simulink library "HEV_Battery_Det_Lib"  (R2017a)
settings: Solver=ode45  StartTime=0.0  StopTime=0.1  RelTol=1e-3  EnableMultiTasking=on
undefined symbols (not defined in the file): BCell_R, HEV_Param, Hydride, Metal, Nickel
libraries: fl_lib x48, nesl_utility x32, Battery_Cell_Det x10, powerlib x8, elec_lib x3, HEV_Battery_Det_Lib x1, Capacitors_lib x1, electricdrivelib x1
Description:
  | Copyright 2014-2017 The MathWorks, Inc.
settings Model: Creator=smiller  LastModifiedBy=smiller
settings DataIOCC: LimitDataPoints=on  SaveFormat=Array  SignalLoggingSaveFormat=ModelDataLogs
settings OptimizationCC: ExpressionDepthLimit=2147483647  LifeSpan=inf
settings DebuggingCC: UnderspecifiedInitializationDetection=Classic  MergeDetectMultiDrivingBlocksExec=none  SolverPrmCheckMsg=warning  FcnCallInpInsideContextMsg=warning  AllowSymbolicDim=off  StateNameClashWarn=warning  SFUnexpectedBacktrackingDiag=warning  SFNoUnconditionalDefaultTransitionDiag=warning  SFExecutionAtInitializationDiag=none
settings HardwareCC: ProdBitPerPointer=32  ProdBitPerSizeT=32  ProdBitPerPtrDiffT=32  ProdLargestAtomicFloat=None  ProdIntDivRoundTo=Undefined  ProdEndianess=Unspecified  ProdWordSize=32  ProdHWDeviceType=32-bit Generic
settings ModelReferenceCC: PropagateSignalLabelsOutOfModel=off
settings GRTTargetCC: TargetLangStandard=C89/C90 (ANSI)  GeneratePreprocessorConditionals=Disable all  CombineOutputUpdateFcns=off  GRTInterface=on
settings ConfigComp: CovMetricSettings=dw  CovHtmlReporting=on  CovSaveCumulativeToWorkspaceVar=on  CovSaveSingleToWorkspaceVar=on  CovExternalEMLEnable=off  CovSFcnEnable=off

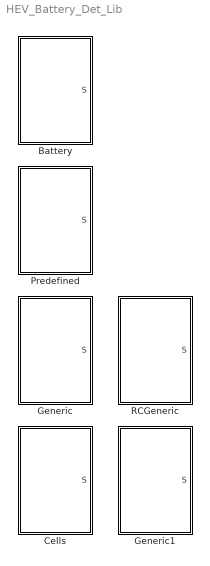
== system HEV_Battery_Det_Lib ==
  Battery : Subsystem  BlockChoice=Generic
      mask init:
      | %disp('Battery Mask Init');
      | %Configure_HEV_Simulation;
      settings: TemplateBlock=self  MemberBlocks=Generic,Predefined
  Cells : Subsystem
      mask Display:
      | image(imread('HEV_Battery_Cells_IMAGE.jpg'));
      | port_label('LConn',1,'+');
      | port_label('LConn',2,'-');
      | port_label('output',1,'S');
  Generic : Subsystem
      mask Display:
      | image(imread('HEV_Battery_Custom_IMAGE.jpg'));
      | port_label('LConn',1,'+');
      | port_label('LConn',2,'-');
      | port_label('output',1,'S');
  Generic1 : Subsystem
      mask Display:
      | image(imread('HEV_Battery_Generic_IMAGE.jpg'));
      | port_label('LConn',1,'+');
      | port_label('LConn',2,'-');
      | port_label('output',1,'S');
  Predefined : Subsystem
      mask Display:
      | image(imread('HEV_Battery_Detailed_IMAGE.jpg'));
      | port_label('LConn',1,'+');
      | port_label('LConn',2,'-');
      | port_label('output',1,'S');
  RCGeneric : Subsystem
      mask Display:
      | image(imread('HEV_Battery_GenericRC_IMAGE.jpg'));
      | port_label('LConn',1,'+');
      | port_label('LConn',2,'-');
      | port_label('output',1,'S');

== system HEV_Battery_Det_Lib/Battery ==
  Generic : HEV_Battery_Det_Lib/Generic  SystemSampleTime=-1
  + : PMIOPort  Port=1  Side=Left
  - : PMIOPort  Port=2  Side=Left
  S : Outport
  wires:
  Generic/1 -> S/1
  connections:
  Generic/LConn1 -- +/RConn1
  Generic/LConn2 -- -/RConn1

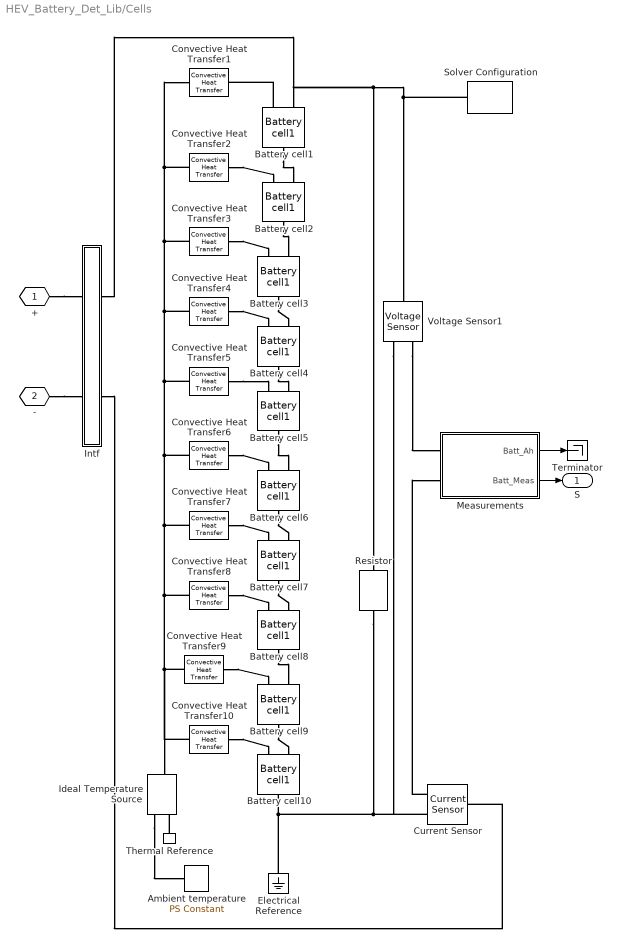
== system HEV_Battery_Det_Lib/Cells ==
  Ambient temperature : fl_lib/Physical Signals/Sources/PS Constant  constant=273+25
  Battery cell{1..10} (10 alike) : Battery_Cell_Det/Battery cell1  SystemSampleTime=-1
  Convective Heat Transfer{1..10} (10 alike) : fl_lib/Thermal/Thermal Elements/Convective Heat Transfer  area=HEV_Param.Battery_Cell.Area m^2  heat_tr_coeff=HEV_Param.Battery_Cell.Rtheta W/(m^2 *K)  Q_specify=off  Q_priority=High  Q=0 J/s  Q_nominal_specify=off  Q_nominal_unit=J/s  Q_nominal_value=1  T_specify=off  T_priority=High  T=0 K  T_nominal_specify=off  T_nominal_unit=K  T_nominal_value=1
  Current Sensor : fl_lib/Electrical/Electrical Sensors/Current Sensor
  Electrical Reference : fl_lib/Electrical/Electrical Elements/Electrical Reference
  Ideal Temperature Source : fl_lib/Thermal/Thermal Sources/Ideal Temperature Source
      settings: SourceProductName=Simscape  SourceProductBaseCode=SS
  Intf : Subsystem  mask(Power Systems ST - Simscape Interface Element){T=100000}
      mask prompts: T "Pole in Transfer Function"
      mask help:
      | Ideal transformer between a Simscape Power Systems ST circuit and a Simscape circuit.
      |
      | The Voltage across the two terminal pairs are equal and the current flowing through the two branches are equal.
      |
      | The coupling has a transfer function and you need to set the pole in the transfer function.
      mask Display:
      | %color('red');
      | %plot([0.3 0.7],[0.775 0.775]);
      | port_label('LConn', 1,'SPS1')
      | port_label('RConn', 1,'SS1')
      | color('black');
      | %plot([0.3 0.7],[0.225 0.225]);
      | port_label('LConn', 2,'SPS2')
      | port_label('RConn', 2,'SS2')
      | %color('green')
      | %text(0.05,0.5,'I Src');
      | %color('blue')
      | %text(0.75,0.5,'V Src');
  Measurements : Subsystem
  Resistor : fl_lib/Electrical/Electrical Elements/Resistor  R=BCell_R Ohm  i_specify=off  i_priority=High  i=0 A  i_nominal_specify=off  i_nominal_unit=A  i_nominal_value=1  v_specify=off  v_priority=High  v=0 V  v_nominal_specify=off  v_nominal_unit=V  v_nominal_value=1
  Solver Configuration : nesl_utility/Solver Configuration  PhysicalDomain=network_engine_domain  SubClassName=solver  LeftPortType=input  RightPortType=generic  Accelerate=off  Tones=[]  Harmonics=[]  SimulateNoise=off  Profile=off  UseLocalSampling=off  EnableSwitchedLinearOptims=on  FrequencyDomain=off  UseCCode=off  RelTol=0.001  AbsTol=1e-06  MinStep=1e-09  ToWorkspace=off  RevertToSquareIcSolve=off  NumHomotopyIterations=100  PhasorMode=off  PhasorModeNumHarmonics=1  OverrideAbsTol=off  DoDC=off  ResidualTolerance=1e-9  UseLocalSolver=off  LocalSolverChoice=NE_BACKWARD_EULER_ADVANCER  LocalSolverSampleTime=.001  DoFixedCost=off  MaxNonlinIter=3  MaxModeIter=2  LinearAlgebra=Sparse  DelaysMemoryBudget=1024  AutomaticFiltering=on  FilteringTimeConstant=0.001
  Terminator : Terminator
  Thermal Reference : fl_lib/Thermal/Thermal Elements/Thermal Reference
  Voltage Sensor1 : fl_lib/Electrical/Electrical Sensors/Voltage Sensor
  + : PMIOPort  Tag=PMCPort  Port=1  Side=Left
  - : PMIOPort  Tag=PMCPort  Port=2  Side=Left
  S : Outport
  wires:
  Measurements/2(Batt_Meas) -> S/1
  Measurements/1(Batt_Ah) -> Terminator/1
  connections:
  Voltage Sensor1/RConn1 -- Measurements/LConn1
  Current Sensor/RConn1 -- Measurements/LConn2
  Intf/RConn2 -- Current Sensor/LConn1
  Voltage Sensor1/RConn2 -- Current Sensor/RConn2 -- Battery cell10/RConn1 -- Electrical Reference/LConn1 -- Resistor/RConn1
  Convective Heat Transfer9/LConn1 -- Convective Heat Transfer10/LConn1 -- Ideal Temperature Source/LConn1 -- Convective Heat Transfer8/LConn1 -- Convective Heat Transfer7/LConn1 -- Convective Heat Transfer6/LConn1 -- Convective Heat Transfer5/LConn1 -- Convective Heat Transfer4/LConn1 -- Convective Heat Transfer3/LConn1 -- Convective Heat Transfer2/LConn1 -- Convective Heat Transfer1/LConn1
  Battery cell1/LConn2 -- Intf/RConn1 -- Voltage Sensor1/LConn1 -- Solver Configuration/RConn1 -- Resistor/LConn1
  Convective Heat Transfer9/RConn1 -- Battery cell9/LConn1
  Battery cell8/RConn1 -- Battery cell9/LConn2
  Convective Heat Transfer8/RConn1 -- Battery cell8/LConn1
  Convective Heat Transfer7/RConn1 -- Battery cell7/LConn1
  Battery cell7/RConn1 -- Battery cell8/LConn2
  Convective Heat Transfer6/RConn1 -- Battery cell6/LConn1
  Battery cell6/RConn1 -- Battery cell7/LConn2
  Battery cell5/RConn1 -- Battery cell6/LConn2
  Convective Heat Transfer5/RConn1 -- Battery cell5/LConn1
  Battery cell4/RConn1 -- Battery cell5/LConn2
  Convective Heat Transfer4/RConn1 -- Battery cell4/LConn1
  Battery cell3/RConn1 -- Battery cell4/LConn2
  Convective Heat Transfer3/RConn1 -- Battery cell3/LConn1
  Battery cell2/RConn1 -- Battery cell3/LConn2
  Battery cell9/RConn1 -- Battery cell10/LConn2
  Convective Heat Transfer2/RConn1 -- Battery cell2/LConn1
  Convective Heat Transfer10/RConn1 -- Battery cell10/LConn1
  Battery cell1/RConn1 -- Battery cell2/LConn2
  Battery cell1/LConn1 -- Convective Heat Transfer1/RConn1
  Ideal Temperature Source/RConn1 -- Ambient temperature/RConn1
  Thermal Reference/LConn1 -- Ideal Temperature Source/RConn2
  +/RConn1 -- Intf/LConn1
  -/RConn1 -- Intf/LConn2

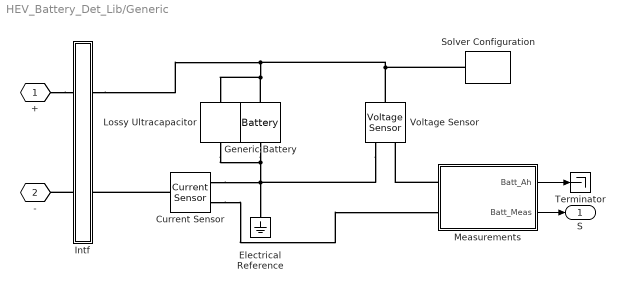
== system HEV_Battery_Det_Lib/Generic ==
  Current Sensor : fl_lib/Electrical/Electrical Sensors/Current Sensor
  Electrical Reference : fl_lib/Electrical/Electrical Elements/Electrical Reference
  Generic Battery : elec_lib/Sources/Battery  Vnom=HEV_Param.Battery_Sys.Nominal_Voltage V  R1=HEV_Param.Battery_Sys.Internal_Resistance Ohm  prm_AH=2  AH=HEV_Param.Battery_Sys.Rated_Capacity hr*A  V1=HEV_Param.Battery_Sys.Expn_Voltage V  AH1=HEV_Param.Battery_Sys.Expn_Charge hr*A  prm_R2=1  R2=2e+3 Ohm  prm_fade=1  N_fade=100  AH_fade=45 hr*A  R1_fade=2.02 Ohm  V1_fade=10.35 V  i_specify=off  i_priority=None  i=0 A  i_nominal_specify=off  i_nominal_unit=A  i_nominal_value=1  v_specify=off  v_priority=None  v=0 V  v_nominal_specify=off  v_nominal_unit=V  v_nominal_value=1  charge_specify=on  charge_priority=High  charge=HEV_Param.Battery_Sys.Initial_Charge hr*A  charge_nominal_specify=off  charge_nominal_unit=hr*A  charge_nominal_value=1  num_cycles_specify=off  num_cycles_priority=High  num_cycles=0  num_cycles_nominal_specify=off  num_cycles_nominal_unit=1  num_cycles_nominal_value=1  thermal_mass=30000 J/K  Tmeas=298.15 K  Vnom_T2=12 V  R1_T2=2.2 Ohm  V1_T2=11.4 V  R2_T2=2200 Ohm  Tmeas2=273.15 K  temperature_specify=off  temperature_priority=High  temperature=298.15 K  temperature_nominal_specify=off  temperature_nominal_unit=K  temperature_nominal_value=1
      settings: SourceProductName=Simscape Electronics  SourceProductBaseCode=SN
  Intf : Subsystem  mask(Power Systems ST - Simscape Interface Element){T=100000}
      mask prompts: T "Pole in Transfer Function"
      mask help:
      | Ideal transformer between a Simscape Power Systems ST circuit and a Simscape circuit.
      |
      | The Voltage across the two terminal pairs are equal and the current flowing through the two branches are equal.
      |
      | The coupling has a transfer function and you need to set the pole in the transfer function.
      mask Display:
      | %color('red');
      | %plot([0.3 0.7],[0.775 0.775]);
      | port_label('LConn', 1,'SPS1')
      | port_label('RConn', 1,'SS1')
      | color('black');
      | %plot([0.3 0.7],[0.225 0.225]);
      | port_label('LConn', 2,'SPS2')
      | port_label('RConn', 2,'SS2')
      | %color('green')
      | %text(0.05,0.5,'I Src');
      | %color('blue')
      | %text(0.75,0.5,'V Src');
  Lossy Ultracapacitor : Capacitors_lib/Lossy Ultracapacitor  C0=HEV_Param.UltraCapacitor.Nominal_Capacitance F  Cv=HEV_Param.UltraCapacitor.Rate_C_V F/V  R=HEV_Param.UltraCapacitor.Series_R Ohm  Rd=HEV_Param.UltraCapacitor.Self_Discharge_R Ohm  i_specify=off  i_priority=High  i=0 A  i_nominal_specify=off  i_nominal_unit=A  i_nominal_value=1  vc_specify=off  vc_priority=High  vc=0 V  vc_nominal_specify=off  vc_nominal_unit=V  vc_nominal_value=1
  Measurements : Subsystem
  Solver Configuration : nesl_utility/Solver Configuration  PhysicalDomain=network_engine_domain  SubClassName=solver  LeftPortType=input  RightPortType=generic  Accelerate=off  Tones=[]  Harmonics=[]  SimulateNoise=off  Profile=off  UseLocalSampling=off  EnableSwitchedLinearOptims=on  FrequencyDomain=off  UseCCode=off  RelTol=0.001  AbsTol=1e-06  MinStep=1e-09  ToWorkspace=off  RevertToSquareIcSolve=off  NumHomotopyIterations=100  PhasorMode=off  PhasorModeNumHarmonics=1  OverrideAbsTol=off  DoDC=off  ResidualTolerance=1e-9  UseLocalSolver=off  LocalSolverChoice=NE_BACKWARD_EULER_ADVANCER  LocalSolverSampleTime=.001  DoFixedCost=off  MaxNonlinIter=3  MaxModeIter=2  LinearAlgebra=Sparse  DelaysMemoryBudget=1024  AutomaticFiltering=on  FilteringTimeConstant=0.001
  Terminator : Terminator
  Voltage Sensor : fl_lib/Electrical/Electrical Sensors/Voltage Sensor
  + : PMIOPort  Tag=PMCPort  Port=1  Side=Left
  - : PMIOPort  Tag=PMCPort  Port=2  Side=Left
  S : Outport
  wires:
  Measurements/1(Batt_Ah) -> Terminator/1
  Measurements/2(Batt_Meas) -> S/1
  connections:
  Measurements/LConn1 -- Voltage Sensor/RConn1
  Intf/RConn1 -- Voltage Sensor/LConn1 -- Solver Configuration/RConn1 -- Generic Battery/LConn1 -- Lossy Ultracapacitor/LConn1
  Generic Battery/RConn1 -- Voltage Sensor/RConn2 -- Electrical Reference/LConn1 -- Current Sensor/RConn2 -- Lossy Ultracapacitor/RConn1
  Current Sensor/RConn1 -- Measurements/LConn2
  Intf/LConn2 -- -/RConn1
  +/RConn1 -- Intf/LConn1
  Current Sensor/LConn1 -- Intf/RConn2

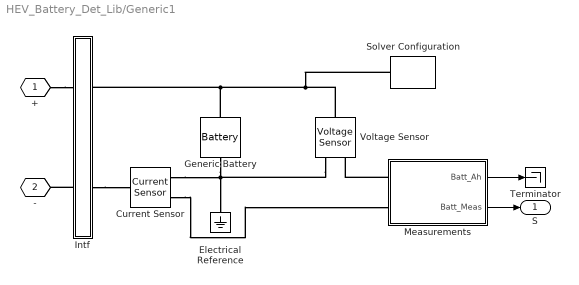
== system HEV_Battery_Det_Lib/Generic1 ==
  Current Sensor : fl_lib/Electrical/Electrical Sensors/Current Sensor
  Electrical Reference : fl_lib/Electrical/Electrical Elements/Electrical Reference
  Generic Battery : elec_lib/Sources/Battery  Vnom=HEV_Param.Battery_Sys.Nominal_Voltage V  R1=HEV_Param.Battery_Sys.Internal_Resistance Ohm  prm_AH=2  AH=HEV_Param.Battery_Sys.Rated_Capacity hr*A  V1=HEV_Param.Battery_Sys.Expn_Voltage V  AH1=HEV_Param.Battery_Sys.Expn_Charge hr*A  prm_R2=1  R2=2e+3 Ohm  prm_fade=1  N_fade=100  AH_fade=45 hr*A  R1_fade=2.02 Ohm  V1_fade=10.35 V  i_specify=off  i_priority=None  i=0 A  i_nominal_specify=off  i_nominal_unit=A  i_nominal_value=1  v_specify=off  v_priority=None  v=0 V  v_nominal_specify=off  v_nominal_unit=V  v_nominal_value=1  charge_specify=on  charge_priority=High  charge=HEV_Param.Battery_Sys.Initial_Charge hr*A  charge_nominal_specify=off  charge_nominal_unit=hr*A  charge_nominal_value=1  num_cycles_specify=off  num_cycles_priority=High  num_cycles=0  num_cycles_nominal_specify=off  num_cycles_nominal_unit=1  num_cycles_nominal_value=1  thermal_mass=30000 J/K  Tmeas=298.15 K  Vnom_T2=12 V  R1_T2=2.2 Ohm  V1_T2=11.4 V  R2_T2=2200 Ohm  Tmeas2=273.15 K  temperature_specify=off  temperature_priority=High  temperature=298.15 K  temperature_nominal_specify=off  temperature_nominal_unit=K  temperature_nominal_value=1
      settings: SourceProductName=Simscape Electronics  SourceProductBaseCode=SN
  Intf : Subsystem  mask(Power Systems ST - Simscape Interface Element){T=100000}
      mask prompts: T "Pole in Transfer Function"
      mask help:
      | Ideal transformer between a Simscape Power Systems ST circuit and a Simscape circuit.
      |
      | The Voltage across the two terminal pairs are equal and the current flowing through the two branches are equal.
      |
      | The coupling has a transfer function and you need to set the pole in the transfer function.
      mask Display:
      | %color('red');
      | %plot([0.3 0.7],[0.775 0.775]);
      | port_label('LConn', 1,'SPS1')
      | port_label('RConn', 1,'SS1')
      | color('black');
      | %plot([0.3 0.7],[0.225 0.225]);
      | port_label('LConn', 2,'SPS2')
      | port_label('RConn', 2,'SS2')
      | %color('green')
      | %text(0.05,0.5,'I Src');
      | %color('blue')
      | %text(0.75,0.5,'V Src');
  Measurements : Subsystem
  Solver Configuration : nesl_utility/Solver Configuration  PhysicalDomain=network_engine_domain  SubClassName=solver  LeftPortType=input  RightPortType=generic  Accelerate=off  Tones=[]  Harmonics=[]  SimulateNoise=off  Profile=off  UseLocalSampling=off  EnableSwitchedLinearOptims=on  FrequencyDomain=off  UseCCode=off  RelTol=0.001  AbsTol=1e-06  MinStep=1e-09  ToWorkspace=off  RevertToSquareIcSolve=off  NumHomotopyIterations=100  PhasorMode=off  PhasorModeNumHarmonics=1  OverrideAbsTol=off  DoDC=off  ResidualTolerance=1e-9  UseLocalSolver=off  LocalSolverChoice=NE_BACKWARD_EULER_ADVANCER  LocalSolverSampleTime=.001  DoFixedCost=off  MaxNonlinIter=3  MaxModeIter=2  LinearAlgebra=Sparse  DelaysMemoryBudget=1024  AutomaticFiltering=on  FilteringTimeConstant=0.001
  Terminator : Terminator
  Voltage Sensor : fl_lib/Electrical/Electrical Sensors/Voltage Sensor
  + : PMIOPort  Tag=PMCPort  Port=1  Side=Left
  - : PMIOPort  Tag=PMCPort  Port=2  Side=Left
  S : Outport
  wires:
  Measurements/2(Batt_Meas) -> S/1
  Measurements/1(Batt_Ah) -> Terminator/1
  connections:
  Intf/RConn2 -- Current Sensor/LConn1
  Current Sensor/RConn1 -- Measurements/LConn2
  Current Sensor/RConn2 -- Electrical Reference/LConn1 -- Generic Battery/RConn1 -- Voltage Sensor/RConn2
  Intf/RConn1 -- Voltage Sensor/LConn1 -- Solver Configuration/RConn1 -- Generic Battery/LConn1
  Measurements/LConn1 -- Voltage Sensor/RConn1
  +/RConn1 -- Intf/LConn1
  Intf/LConn2 -- -/RConn1

== system HEV_Battery_Det_Lib/Predefined ==
  GF1 : Subsystem
      mask Display: disp('GF')
  Preset Battery : electricdrivelib/Extra Sources/Battery  BatType=Nickel-Metal-Hydride  ShowTempParam=off  ThermalPreset=no  ShowAgeParam=off  NomV=HEV_Param.Battery_Det.Nominal_Voltage  NomQ=HEV_Param.Battery_Det.Rated_Capacity  SOC=HEV_Param.Battery_Det.Initial_SOC  Batt_Tr=30  PresetModel=on  MaxQ=8.7231  MinV=150  FullV=235.5932  Dis_rate=1.62  R=0.24691  Normal_OP=7.7885  expZone="[216.9492          1.62]"  current=[50 100]  Units=Time  Tci=20  NomT=20  T2=-30  MaxQ2=4.8  FullV2=7.1  Normal_OP2=5.72  expZone2="[6.58  1]"  Rca=0.6  ti=1000  Dp=0  Neq0=0  Tsim=1e6  Ta1=25  Qeol=5.4*0.9  Reol=0.013333*1.2  Char_age=[2.3478, 3]  Dis_age=[2.3478, 10]  N1=1500  N2=10500  N3=1000  N4=1400  Ta2=45  N5=950
  + : PMIOPort  Tag=PMCPort  Port=1  Side=Left
  - : PMIOPort  Tag=PMCPort  Port=2  Side=Left
  S : Outport
  wires:
  Preset Battery/1 -> GF1/1(In1)
  GF1/1(Out1) -> S/1
  connections:
  +/RConn1 -- Preset Battery/LConn1
  Preset Battery/LConn2 -- -/RConn1

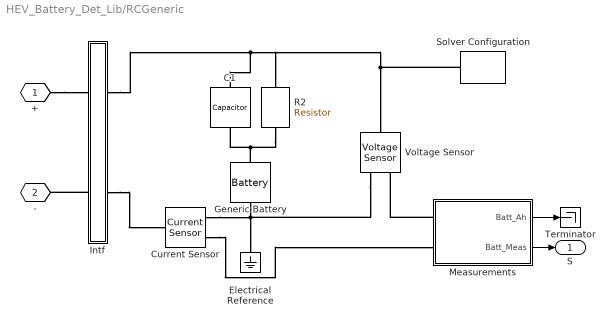
== system HEV_Battery_Det_Lib/RCGeneric ==
  C1 : fl_lib/Electrical/Electrical Elements/Capacitor  c=HEV_Param.Battery_Sys.C1.Capacitance F  r=HEV_Param.Battery_Sys.C1.Series_Resistance Ohm  g=0 1/Ohm  i_specify=off  i_priority=High  i=0 A  i_nominal_specify=off  i_nominal_unit=A  i_nominal_value=1  v_specify=off  v_priority=High  v=0 V  v_nominal_specify=off  v_nominal_unit=V  v_nominal_value=1  vc_specify=on  vc_priority=High  vc=HEV_Param.Battery_Sys.C1.Initial_Voltage V  vc_nominal_specify=off  vc_nominal_unit=V  vc_nominal_value=1
  Current Sensor : fl_lib/Electrical/Electrical Sensors/Current Sensor
  Electrical Reference : fl_lib/Electrical/Electrical Elements/Electrical Reference
  Generic Battery : elec_lib/Sources/Battery  Vnom=HEV_Param.Battery_Sys.Nominal_Voltage V  R1=HEV_Param.Battery_Sys.Internal_Resistance Ohm  prm_AH=2  AH=HEV_Param.Battery_Sys.Rated_Capacity hr*A  V1=HEV_Param.Battery_Sys.Expn_Voltage V  AH1=HEV_Param.Battery_Sys.Expn_Charge hr*A  prm_R2=1  R2=2e+3 Ohm  prm_fade=1  N_fade=100  AH_fade=45 hr*A  R1_fade=2.02 Ohm  V1_fade=10.35 V  i_specify=off  i_priority=None  i=0 A  i_nominal_specify=off  i_nominal_unit=A  i_nominal_value=1  v_specify=off  v_priority=None  v=0 V  v_nominal_specify=off  v_nominal_unit=V  v_nominal_value=1  charge_specify=on  charge_priority=High  charge=HEV_Param.Battery_Sys.Initial_Charge hr*A  charge_nominal_specify=off  charge_nominal_unit=hr*A  charge_nominal_value=1  num_cycles_specify=off  num_cycles_priority=High  num_cycles=0  num_cycles_nominal_specify=off  num_cycles_nominal_unit=1  num_cycles_nominal_value=1  thermal_mass=30000 J/K  Tmeas=298.15 K  Vnom_T2=12 V  R1_T2=2.2 Ohm  V1_T2=11.4 V  R2_T2=2200 Ohm  Tmeas2=273.15 K  temperature_specify=off  temperature_priority=High  temperature=298.15 K  temperature_nominal_specify=off  temperature_nominal_unit=K  temperature_nominal_value=1
      settings: SourceProductName=Simscape Electronics  SourceProductBaseCode=SN
  Intf : Subsystem  mask(Power Systems ST - Simscape Interface Element){T=100000}
      mask prompts: T "Pole in Transfer Function"
      mask help:
      | Ideal transformer between a Simscape Power Systems ST circuit and a Simscape circuit.
      |
      | The Voltage across the two terminal pairs are equal and the current flowing through the two branches are equal.
      |
      | The coupling has a transfer function and you need to set the pole in the transfer function.
      mask Display:
      | %color('red');
      | %plot([0.3 0.7],[0.775 0.775]);
      | port_label('LConn', 1,'SPS1')
      | port_label('RConn', 1,'SS1')
      | color('black');
      | %plot([0.3 0.7],[0.225 0.225]);
      | port_label('LConn', 2,'SPS2')
      | port_label('RConn', 2,'SS2')
      | %color('green')
      | %text(0.05,0.5,'I Src');
      | %color('blue')
      | %text(0.75,0.5,'V Src');
  Measurements : Subsystem
  R2 : fl_lib/Electrical/Electrical Elements/Resistor  R=HEV_Param.Battery_Sys.R2 Ohm  i_specify=off  i_priority=High  i=0 A  i_nominal_specify=off  i_nominal_unit=A  i_nominal_value=1  v_specify=off  v_priority=High  v=0 V  v_nominal_specify=off  v_nominal_unit=V  v_nominal_value=1
  Solver Configuration : nesl_utility/Solver Configuration  PhysicalDomain=network_engine_domain  SubClassName=solver  LeftPortType=input  RightPortType=generic  Accelerate=off  Tones=[]  Harmonics=[]  SimulateNoise=off  Profile=off  UseLocalSampling=off  EnableSwitchedLinearOptims=on  FrequencyDomain=off  UseCCode=off  RelTol=0.001  AbsTol=1e-06  MinStep=1e-09  ToWorkspace=off  RevertToSquareIcSolve=off  NumHomotopyIterations=100  PhasorMode=off  PhasorModeNumHarmonics=1  OverrideAbsTol=off  DoDC=off  ResidualTolerance=1e-9  UseLocalSolver=off  LocalSolverChoice=NE_BACKWARD_EULER_ADVANCER  LocalSolverSampleTime=.001  DoFixedCost=off  MaxNonlinIter=3  MaxModeIter=2  LinearAlgebra=Sparse  DelaysMemoryBudget=1024  AutomaticFiltering=on  FilteringTimeConstant=0.001
  Terminator : Terminator
  Voltage Sensor : fl_lib/Electrical/Electrical Sensors/Voltage Sensor
  + : PMIOPort  Tag=PMCPort  Port=1  Side=Left
  - : PMIOPort  Tag=PMCPort  Port=2  Side=Left
  S : Outport
  wires:
  Measurements/1(Batt_Ah) -> Terminator/1
  Measurements/2(Batt_Meas) -> S/1
  connections:
  Measurements/LConn1 -- Voltage Sensor/RConn1
  Intf/RConn1 -- Voltage Sensor/LConn1 -- Solver Configuration/RConn1 -- R2/LConn1 -- C1/LConn1
  Voltage Sensor/RConn2 -- Generic Battery/RConn1 -- Electrical Reference/LConn1 -- Current Sensor/RConn2
  Current Sensor/RConn1 -- Measurements/LConn2
  Intf/RConn2 -- Current Sensor/LConn1
  Generic Battery/LConn1 -- R2/RConn1 -- C1/RConn1
  +/RConn1 -- Intf/LConn1
  Intf/LConn2 -- -/RConn1

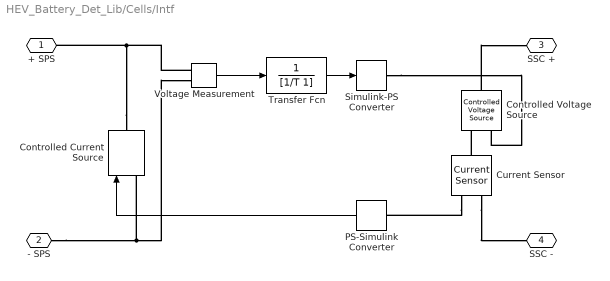
== system HEV_Battery_Det_Lib/Cells/Intf ==
  Controlled Voltage Source : fl_lib/Electrical/Electrical Sources/Controlled Voltage Source
  Controlled Current Source : powerlib/Electrical Sources/Controlled Current Source  Initialize=on  Source_Type=AC  Amplitude=0  Phase=0  Frequency=0  Measurements=None
  Current Sensor : fl_lib/Electrical/Electrical Sensors/Current Sensor
  PS-Simulink Converter : nesl_utility/PS-Simulink Converter  PhysicalDomain=network_engine_domain  SubClassName=ps_output  LeftPortType=input  RightPortType=output  PseudoPeriodic=off  Frequencies=[]  Unit=A  AffineConversion=off
  Simulink-PS Converter : nesl_utility/Simulink-PS Converter  PhysicalDomain=network_engine_domain  SubClassName=ps_input  LeftPortType=input  RightPortType=output  PseudoPeriodic=off  Frequencies=[]  NoiseDistribution=none  NoiseParameters=[]  Unit=V  AffineConversion=off  FilteringAndDerivatives=zero  SimscapeFilterOrder=1  InputFilterTimeConstant=.001  UdotUserProvided=0
  Transfer Fcn : TransferFcn  Denominator=[1/T 1]
  Voltage Measurement : powerlib/Measurements/Voltage Measurement  PhasorSimulation=off  OutputType=Complex  PSBequivalent=0
  + SPS : PMIOPort  Port=1  Side=Left
  - SPS : PMIOPort  Port=2  Side=Left
  SSC + : PMIOPort  Port=3  Side=Right
  SSC - : PMIOPort  Port=4  Side=Right
  wires:
  PS-Simulink Converter/1 -> Controlled Current Source/1
  Voltage Measurement/1 -> Transfer Fcn/1
  Transfer Fcn/1 -> Simulink-PS Converter/1
  connections:
  Controlled Voltage Source/LConn1 -- SSC +/RConn1
  Current Sensor/LConn1 -- Controlled Voltage Source/RConn2
  Simulink-PS Converter/RConn1 -- Controlled Voltage Source/RConn1
  Current Sensor/RConn1 -- PS-Simulink Converter/LConn1
  Controlled Current Source/LConn1 -- Voltage Measurement/LConn2 -- - SPS/RConn1
  Current Sensor/RConn2 -- SSC -/RConn1
  Controlled Current Source/RConn1 -- + SPS/RConn1 -- Voltage Measurement/LConn1

== system HEV_Battery_Det_Lib/Cells/Measurements ==
  Bus Creator : BusCreator  Inputs=4
  Calc Pct : Gain  Gain=1/HEV_Param.Battery_Sys.Maximum_Capacity*100
  Calculate battery power & charge : Subsystem
  PS-Simulink Converter1 : nesl_utility/PS-Simulink Converter  PhysicalDomain=network_engine_domain  SubClassName=ps_output  LeftPortType=input  RightPortType=output  PseudoPeriodic=off  Frequencies=[]  Unit=V  AffineConversion=off
  PS-Simulink Converter2 : nesl_utility/PS-Simulink Converter  PhysicalDomain=network_engine_domain  SubClassName=ps_output  LeftPortType=input  RightPortType=output  PseudoPeriodic=off  Frequencies=[]  Unit=A  AffineConversion=off
  VBatt : PMIOPort  Port=1  Side=Left
  IBatt : PMIOPort  Port=2  Side=Left
  Batt_Ah : Outport
  Batt_Meas : Outport  Port=2
  tag scope: Batt_Measures=global
  wires:
  Bus Creator/1 -> Batt_Meas/1, [Batt_Measures]
  PS-Simulink Converter2/1 -> Bus Creator/4  "Current (A)"
  PS-Simulink Converter1/1 -> Bus Creator/3  "Voltage (V)"
  Calc Pct/1 -> Bus Creator/2  "SOC (%)"
  Calculate battery power & charge/1(Ah) -> Batt_Ah/1, Calc Pct/1, Bus Creator/1  "Batt_Ah"
  connections:
  PS-Simulink Converter2/LConn1 -- IBatt/RConn1 -- Calculate battery power & charge/LConn2
  PS-Simulink Converter1/LConn1 -- VBatt/RConn1 -- Calculate battery power & charge/LConn1

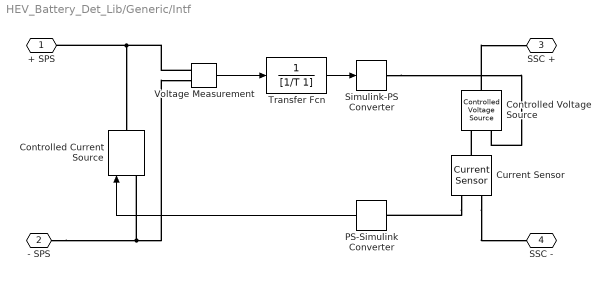
== system HEV_Battery_Det_Lib/Generic/Intf ==
  Controlled Voltage Source : fl_lib/Electrical/Electrical Sources/Controlled Voltage Source
  Controlled Current Source : powerlib/Electrical Sources/Controlled Current Source  Initialize=on  Source_Type=AC  Amplitude=0  Phase=0  Frequency=0  Measurements=None
  Current Sensor : fl_lib/Electrical/Electrical Sensors/Current Sensor
  PS-Simulink Converter : nesl_utility/PS-Simulink Converter  PhysicalDomain=network_engine_domain  SubClassName=ps_output  LeftPortType=input  RightPortType=output  PseudoPeriodic=off  Frequencies=[]  Unit=A  AffineConversion=off
  Simulink-PS Converter : nesl_utility/Simulink-PS Converter  PhysicalDomain=network_engine_domain  SubClassName=ps_input  LeftPortType=input  RightPortType=output  PseudoPeriodic=off  Frequencies=[]  NoiseDistribution=none  NoiseParameters=[]  Unit=V  AffineConversion=off  FilteringAndDerivatives=zero  SimscapeFilterOrder=1  InputFilterTimeConstant=.001  UdotUserProvided=0
  Transfer Fcn : TransferFcn  Denominator=[1/T 1]
  Voltage Measurement : powerlib/Measurements/Voltage Measurement  PhasorSimulation=off  OutputType=Complex  PSBequivalent=0
  + SPS : PMIOPort  Port=1  Side=Left
  - SPS : PMIOPort  Port=2  Side=Left
  SSC + : PMIOPort  Port=3  Side=Right
  SSC - : PMIOPort  Port=4  Side=Right
  wires:
  Transfer Fcn/1 -> Simulink-PS Converter/1
  Voltage Measurement/1 -> Transfer Fcn/1
  PS-Simulink Converter/1 -> Controlled Current Source/1
  connections:
  Voltage Measurement/LConn1 -- + SPS/RConn1 -- Controlled Current Source/RConn1
  Current Sensor/RConn2 -- SSC -/RConn1
  - SPS/RConn1 -- Voltage Measurement/LConn2 -- Controlled Current Source/LConn1
  Current Sensor/RConn1 -- PS-Simulink Converter/LConn1
  Simulink-PS Converter/RConn1 -- Controlled Voltage Source/RConn1
  Current Sensor/LConn1 -- Controlled Voltage Source/RConn2
  Controlled Voltage Source/LConn1 -- SSC +/RConn1

== system HEV_Battery_Det_Lib/Generic/Measurements ==
  Bus Creator : BusCreator  Inputs=4
  Calc Pct : Gain  Gain=1/HEV_Param.Battery_Sys.Maximum_Capacity*100
  Calculate battery power & charge : Subsystem
  PS-Simulink Converter1 : nesl_utility/PS-Simulink Converter  PhysicalDomain=network_engine_domain  SubClassName=ps_output  LeftPortType=input  RightPortType=output  PseudoPeriodic=off  Frequencies=[]  Unit=V  AffineConversion=off
  PS-Simulink Converter2 : nesl_utility/PS-Simulink Converter  PhysicalDomain=network_engine_domain  SubClassName=ps_output  LeftPortType=input  RightPortType=output  PseudoPeriodic=off  Frequencies=[]  Unit=A  AffineConversion=off
  VBatt : PMIOPort  Port=1  Side=Left
  IBatt : PMIOPort  Port=2  Side=Left
  Batt_Ah : Outport
  Batt_Meas : Outport  Port=2
  tag scope: Batt_Measures=global
  wires:
  Bus Creator/1 -> Batt_Meas/1, [Batt_Measures]
  PS-Simulink Converter2/1 -> Bus Creator/4  "Current (A)"
  PS-Simulink Converter1/1 -> Bus Creator/3  "Voltage (V)"
  Calc Pct/1 -> Bus Creator/2  "SOC (%)"
  Calculate battery power & charge/1(Ah) -> Batt_Ah/1, Calc Pct/1, Bus Creator/1  "Batt_Ah"
  connections:
  PS-Simulink Converter2/LConn1 -- IBatt/RConn1 -- Calculate battery power & charge/LConn2
  PS-Simulink Converter1/LConn1 -- VBatt/RConn1 -- Calculate battery power & charge/LConn1

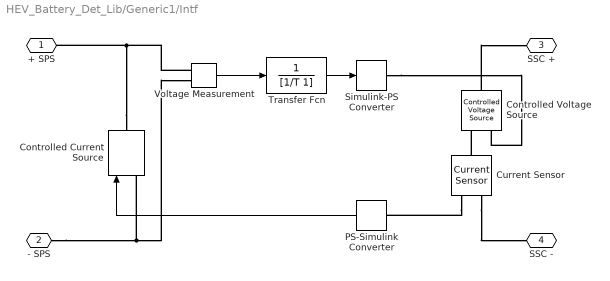
== system HEV_Battery_Det_Lib/Generic1/Intf ==
  Controlled Voltage Source : fl_lib/Electrical/Electrical Sources/Controlled Voltage Source
  Controlled Current Source : powerlib/Electrical Sources/Controlled Current Source  Initialize=on  Source_Type=AC  Amplitude=0  Phase=0  Frequency=0  Measurements=None
  Current Sensor : fl_lib/Electrical/Electrical Sensors/Current Sensor
  PS-Simulink Converter : nesl_utility/PS-Simulink Converter  PhysicalDomain=network_engine_domain  SubClassName=ps_output  LeftPortType=input  RightPortType=output  PseudoPeriodic=off  Frequencies=[]  Unit=A  AffineConversion=off
  Simulink-PS Converter : nesl_utility/Simulink-PS Converter  PhysicalDomain=network_engine_domain  SubClassName=ps_input  LeftPortType=input  RightPortType=output  PseudoPeriodic=off  Frequencies=[]  NoiseDistribution=none  NoiseParameters=[]  Unit=V  AffineConversion=off  FilteringAndDerivatives=zero  SimscapeFilterOrder=1  InputFilterTimeConstant=.001  UdotUserProvided=0
  Transfer Fcn : TransferFcn  Denominator=[1/T 1]
  Voltage Measurement : powerlib/Measurements/Voltage Measurement  PhasorSimulation=off  OutputType=Complex  PSBequivalent=0
  + SPS : PMIOPort  Port=1  Side=Left
  - SPS : PMIOPort  Port=2  Side=Left
  SSC + : PMIOPort  Port=3  Side=Right
  SSC - : PMIOPort  Port=4  Side=Right
  wires:
  PS-Simulink Converter/1 -> Controlled Current Source/1
  Voltage Measurement/1 -> Transfer Fcn/1
  Transfer Fcn/1 -> Simulink-PS Converter/1
  connections:
  Controlled Voltage Source/LConn1 -- SSC +/RConn1
  Current Sensor/LConn1 -- Controlled Voltage Source/RConn2
  Simulink-PS Converter/RConn1 -- Controlled Voltage Source/RConn1
  Current Sensor/RConn1 -- PS-Simulink Converter/LConn1
  Controlled Current Source/LConn1 -- Voltage Measurement/LConn2 -- - SPS/RConn1
  Current Sensor/RConn2 -- SSC -/RConn1
  Controlled Current Source/RConn1 -- + SPS/RConn1 -- Voltage Measurement/LConn1

== system HEV_Battery_Det_Lib/Generic1/Measurements ==
  Bus Creator : BusCreator  Inputs=4
  Calc Pct : Gain  Gain=1/HEV_Param.Battery_Sys.Maximum_Capacity*100
  Calculate battery power & charge : Subsystem
  PS-Simulink Converter1 : nesl_utility/PS-Simulink Converter  PhysicalDomain=network_engine_domain  SubClassName=ps_output  LeftPortType=input  RightPortType=output  PseudoPeriodic=off  Frequencies=[]  Unit=V  AffineConversion=off
  PS-Simulink Converter2 : nesl_utility/PS-Simulink Converter  PhysicalDomain=network_engine_domain  SubClassName=ps_output  LeftPortType=input  RightPortType=output  PseudoPeriodic=off  Frequencies=[]  Unit=A  AffineConversion=off
  VBatt : PMIOPort  Port=1  Side=Left
  IBatt : PMIOPort  Port=2  Side=Left
  Batt_Ah : Outport
  Batt_Meas : Outport  Port=2
  tag scope: Batt_Measures=global
  wires:
  Calculate battery power & charge/1(Ah) -> Bus Creator/1, Calc Pct/1, Batt_Ah/1  "Batt_Ah"
  Calc Pct/1 -> Bus Creator/2  "SOC (%)"
  PS-Simulink Converter1/1 -> Bus Creator/3  "Voltage (V)"
  PS-Simulink Converter2/1 -> Bus Creator/4  "Current (A)"
  Bus Creator/1 -> [Batt_Measures], Batt_Meas/1
  connections:
  Calculate battery power & charge/LConn1 -- VBatt/RConn1 -- PS-Simulink Converter1/LConn1
  Calculate battery power & charge/LConn2 -- IBatt/RConn1 -- PS-Simulink Converter2/LConn1

== system HEV_Battery_Det_Lib/Predefined/GF1 ==
  In1 : Inport
  SOC Offset : Subsystem
      mask Display: disp('A')
  Out1 : Outport
  tag scope: Batt_Measures=global
  wires:
  In1/1 -> SOC Offset/1(In1)
  SOC Offset/1(Out1) -> [Batt_Measures], Out1/1

== system HEV_Battery_Det_Lib/RCGeneric/Intf ==
  Controlled Voltage Source : fl_lib/Electrical/Electrical Sources/Controlled Voltage Source
  Controlled Current Source : powerlib/Electrical Sources/Controlled Current Source  Initialize=on  Source_Type=AC  Amplitude=0  Phase=0  Frequency=0  Measurements=None
  Current Sensor : fl_lib/Electrical/Electrical Sensors/Current Sensor
  PS-Simulink Converter : nesl_utility/PS-Simulink Converter  PhysicalDomain=network_engine_domain  SubClassName=ps_output  LeftPortType=input  RightPortType=output  PseudoPeriodic=off  Frequencies=[]  Unit=A  AffineConversion=off
  Simulink-PS Converter : nesl_utility/Simulink-PS Converter  PhysicalDomain=network_engine_domain  SubClassName=ps_input  LeftPortType=input  RightPortType=output  PseudoPeriodic=off  Frequencies=[]  NoiseDistribution=none  NoiseParameters=[]  Unit=V  AffineConversion=off  FilteringAndDerivatives=zero  SimscapeFilterOrder=1  InputFilterTimeConstant=.001  UdotUserProvided=0
  Transfer Fcn : TransferFcn  Denominator=[1/T 1]
  Voltage Measurement : powerlib/Measurements/Voltage Measurement  PhasorSimulation=off  OutputType=Complex  PSBequivalent=0
  + SPS : PMIOPort  Port=1  Side=Left
  - SPS : PMIOPort  Port=2  Side=Left
  SSC + : PMIOPort  Port=3  Side=Right
  SSC - : PMIOPort  Port=4  Side=Right
  wires:
  PS-Simulink Converter/1 -> Controlled Current Source/1
  Voltage Measurement/1 -> Transfer Fcn/1
  Transfer Fcn/1 -> Simulink-PS Converter/1
  connections:
  Controlled Voltage Source/LConn1 -- SSC +/RConn1
  Current Sensor/LConn1 -- Controlled Voltage Source/RConn2
  Simulink-PS Converter/RConn1 -- Controlled Voltage Source/RConn1
  Current Sensor/RConn1 -- PS-Simulink Converter/LConn1
  Controlled Current Source/LConn1 -- Voltage Measurement/LConn2 -- - SPS/RConn1
  Current Sensor/RConn2 -- SSC -/RConn1
  Controlled Current Source/RConn1 -- + SPS/RConn1 -- Voltage Measurement/LConn1

== system HEV_Battery_Det_Lib/RCGeneric/Measurements ==
  Bus Creator : BusCreator  Inputs=4
  Calc Pct : Gain  Gain=1/HEV_Param.Battery_Sys.Maximum_Capacity*100
  Calculate battery power & charge : Subsystem
  PS-Simulink Converter1 : nesl_utility/PS-Simulink Converter  PhysicalDomain=network_engine_domain  SubClassName=ps_output  LeftPortType=input  RightPortType=output  PseudoPeriodic=off  Frequencies=[]  Unit=V  AffineConversion=off
  PS-Simulink Converter2 : nesl_utility/PS-Simulink Converter  PhysicalDomain=network_engine_domain  SubClassName=ps_output  LeftPortType=input  RightPortType=output  PseudoPeriodic=off  Frequencies=[]  Unit=A  AffineConversion=off
  VBatt : PMIOPort  Port=1  Side=Left
  IBatt : PMIOPort  Port=2  Side=Left
  Batt_Ah : Outport
  Batt_Meas : Outport  Port=2
  tag scope: Batt_Measures=global
  wires:
  Bus Creator/1 -> Batt_Meas/1, [Batt_Measures]
  PS-Simulink Converter2/1 -> Bus Creator/4  "Current (A)"
  PS-Simulink Converter1/1 -> Bus Creator/3  "Voltage (V)"
  Calc Pct/1 -> Bus Creator/2  "SOC (%)"
  Calculate battery power & charge/1(Ah) -> Batt_Ah/1, Calc Pct/1, Bus Creator/1  "Batt_Ah"
  connections:
  PS-Simulink Converter2/LConn1 -- IBatt/RConn1 -- Calculate battery power & charge/LConn2
  PS-Simulink Converter1/LConn1 -- VBatt/RConn1 -- Calculate battery power & charge/LConn1

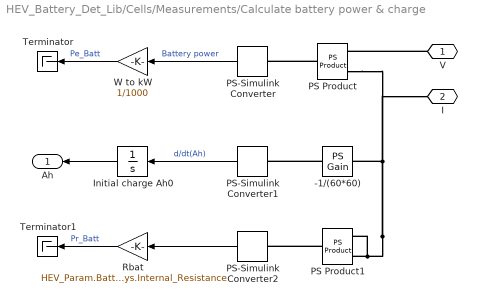
== system HEV_Battery_Det_Lib/Cells/Measurements/Calculate battery power & charge ==
  -1/(60*60) : fl_lib/Physical Signals/Functions/PS Gain  gain=-1/(60*60)
  Initial charge Ah0 : Integrator  InitialCondition=HEV_Param.Battery_Sys.Maximum_Capacity
  PS Product : fl_lib/Physical Signals/Functions/PS Product
      settings: SourceProductName=Simscape
  PS Product1 : fl_lib/Physical Signals/Functions/PS Product
      settings: SourceProductName=Simscape
  PS-Simulink Converter : nesl_utility/PS-Simulink Converter  PhysicalDomain=network_engine_domain  SubClassName=ps_output  LeftPortType=input  RightPortType=output  PseudoPeriodic=off  Frequencies=[]  Unit=W  AffineConversion=off
  PS-Simulink Converter1 : nesl_utility/PS-Simulink Converter  PhysicalDomain=network_engine_domain  SubClassName=ps_output  LeftPortType=input  RightPortType=output  PseudoPeriodic=off  Frequencies=[]  Unit=1  AffineConversion=off
  PS-Simulink Converter2 : nesl_utility/PS-Simulink Converter  PhysicalDomain=network_engine_domain  SubClassName=ps_output  LeftPortType=input  RightPortType=output  PseudoPeriodic=off  Frequencies=[]  Unit=1  AffineConversion=off
  Rbat : Gain  Gain=HEV_Param.Battery_Sys.Internal_Resistance
  Terminator : Terminator
  Terminator1 : Terminator
  W to kW : Gain  Gain=1/1000
  V : PMIOPort  Port=1  Side=Left
  I : PMIOPort  Port=2  Side=Left
  Ah : Outport
  wires:
  Rbat/1 -> Terminator1/1  "Pr_Batt"
  PS-Simulink Converter2/1 -> Rbat/1
  Initial charge Ah0/1 -> Ah/1
  PS-Simulink Converter1/1 -> Initial charge Ah0/1  "d/dt(Ah)"
  W to kW/1 -> Terminator/1  "Pe_Batt"
  PS-Simulink Converter/1 -> W to kW/1  "Battery power"
  connections:
  PS Product1/RConn1 -- PS-Simulink Converter2/LConn1
  -1/(60*60)/RConn1 -- PS-Simulink Converter1/LConn1
  PS Product1/LConn2 -- PS Product1/LConn1 -- -1/(60*60)/LConn1 -- I/RConn1 -- PS Product/LConn2
  V/RConn1 -- PS Product/LConn1
  PS Product/RConn1 -- PS-Simulink Converter/LConn1

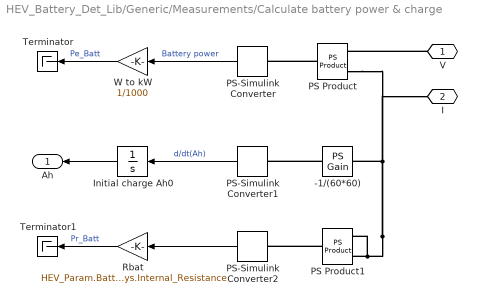
== system HEV_Battery_Det_Lib/Generic/Measurements/Calculate battery power & charge ==
  -1/(60*60) : fl_lib/Physical Signals/Functions/PS Gain  gain=-1/(60*60)
  Initial charge Ah0 : Integrator  InitialCondition=HEV_Param.Battery_Sys.Maximum_Capacity
  PS Product : fl_lib/Physical Signals/Functions/PS Product
      settings: SourceProductName=Simscape
  PS Product1 : fl_lib/Physical Signals/Functions/PS Product
      settings: SourceProductName=Simscape
  PS-Simulink Converter : nesl_utility/PS-Simulink Converter  PhysicalDomain=network_engine_domain  SubClassName=ps_output  LeftPortType=input  RightPortType=output  PseudoPeriodic=off  Frequencies=[]  Unit=W  AffineConversion=off
  PS-Simulink Converter1 : nesl_utility/PS-Simulink Converter  PhysicalDomain=network_engine_domain  SubClassName=ps_output  LeftPortType=input  RightPortType=output  PseudoPeriodic=off  Frequencies=[]  Unit=1  AffineConversion=off
  PS-Simulink Converter2 : nesl_utility/PS-Simulink Converter  PhysicalDomain=network_engine_domain  SubClassName=ps_output  LeftPortType=input  RightPortType=output  PseudoPeriodic=off  Frequencies=[]  Unit=1  AffineConversion=off
  Rbat : Gain  Gain=HEV_Param.Battery_Sys.Internal_Resistance
  Terminator : Terminator
  Terminator1 : Terminator
  W to kW : Gain  Gain=1/1000
  V : PMIOPort  Port=1  Side=Left
  I : PMIOPort  Port=2  Side=Left
  Ah : Outport
  wires:
  Rbat/1 -> Terminator1/1  "Pr_Batt"
  PS-Simulink Converter2/1 -> Rbat/1
  Initial charge Ah0/1 -> Ah/1
  PS-Simulink Converter1/1 -> Initial charge Ah0/1  "d/dt(Ah)"
  W to kW/1 -> Terminator/1  "Pe_Batt"
  PS-Simulink Converter/1 -> W to kW/1  "Battery power"
  connections:
  PS Product1/RConn1 -- PS-Simulink Converter2/LConn1
  -1/(60*60)/RConn1 -- PS-Simulink Converter1/LConn1
  PS Product1/LConn2 -- PS Product1/LConn1 -- -1/(60*60)/LConn1 -- I/RConn1 -- PS Product/LConn2
  V/RConn1 -- PS Product/LConn1
  PS Product/RConn1 -- PS-Simulink Converter/LConn1

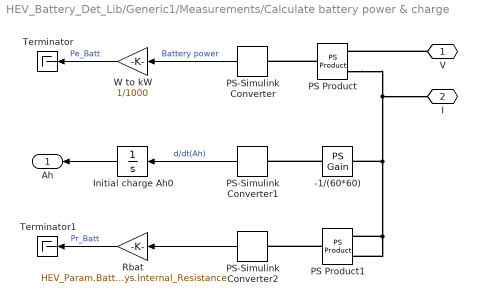
== system HEV_Battery_Det_Lib/Generic1/Measurements/Calculate battery power & charge ==
  -1/(60*60) : fl_lib/Physical Signals/Functions/PS Gain  gain=-1/(60*60)
  Initial charge Ah0 : Integrator  InitialCondition=HEV_Param.Battery_Sys.Maximum_Capacity
  PS Product : fl_lib/Physical Signals/Functions/PS Product
      settings: SourceProductName=Simscape
  PS Product1 : fl_lib/Physical Signals/Functions/PS Product
      settings: SourceProductName=Simscape
  PS-Simulink Converter : nesl_utility/PS-Simulink Converter  PhysicalDomain=network_engine_domain  SubClassName=ps_output  LeftPortType=input  RightPortType=output  PseudoPeriodic=off  Frequencies=[]  Unit=W  AffineConversion=off
  PS-Simulink Converter1 : nesl_utility/PS-Simulink Converter  PhysicalDomain=network_engine_domain  SubClassName=ps_output  LeftPortType=input  RightPortType=output  PseudoPeriodic=off  Frequencies=[]  Unit=1  AffineConversion=off
  PS-Simulink Converter2 : nesl_utility/PS-Simulink Converter  PhysicalDomain=network_engine_domain  SubClassName=ps_output  LeftPortType=input  RightPortType=output  PseudoPeriodic=off  Frequencies=[]  Unit=1  AffineConversion=off
  Rbat : Gain  Gain=HEV_Param.Battery_Sys.Internal_Resistance
  Terminator : Terminator
  Terminator1 : Terminator
  W to kW : Gain  Gain=1/1000
  V : PMIOPort  Port=1  Side=Left
  I : PMIOPort  Port=2  Side=Left
  Ah : Outport
  wires:
  PS-Simulink Converter/1 -> W to kW/1  "Battery power"
  W to kW/1 -> Terminator/1  "Pe_Batt"
  PS-Simulink Converter1/1 -> Initial charge Ah0/1  "d/dt(Ah)"
  Initial charge Ah0/1 -> Ah/1
  PS-Simulink Converter2/1 -> Rbat/1
  Rbat/1 -> Terminator1/1  "Pr_Batt"
  connections:
  PS Product/RConn1 -- PS-Simulink Converter/LConn1
  V/RConn1 -- PS Product/LConn1
  PS Product/LConn2 -- I/RConn1 -- -1/(60*60)/LConn1 -- PS Product1/LConn1 -- PS Product1/LConn2
  -1/(60*60)/RConn1 -- PS-Simulink Converter1/LConn1
  PS Product1/RConn1 -- PS-Simulink Converter2/LConn1

== system HEV_Battery_Det_Lib/Predefined/GF1/SOC Offset ==
  note: For control logic to work consistently
      | for all versions, SOC% must be scaled
  In1 : Inport
  Bus Creator1 : BusCreator  Inputs=4
  Bus Selector : BusSelector  OutputSignals=SOC (%)
  Bus Selector1 : BusSelector  OutputSignals=Current (A),Voltage (V)
  Gain : Gain  Gain=100/HEV_Param.Battery_Det.Initial_SOC
  Gain1 : Gain  Gain=-1/(60*60)
  Initial charge Ah0 : Integrator  InitialCondition=HEV_Param.Battery_Det.Rated_Capacity*HEV_Param.Battery_Det.Initial_SOC/100
  Out1 : Outport
  wires:
  Bus Creator1/1 -> Out1/1
  Bus Selector1/2 -> Bus Creator1/3  "<Voltage (V)>"
  Gain/1 -> Bus Creator1/4  "SOC (%)"
  Bus Selector1/1 -> Bus Creator1/2, Gain1/1  "<Current (A)>"
  Bus Selector/1 -> Gain/1  "<SOC (%)>"
  In1/1 -> Bus Selector1/1, Bus Selector/1
  Gain1/1 -> Initial charge Ah0/1
  Initial charge Ah0/1 -> Bus Creator1/1  "Batt_Ah"

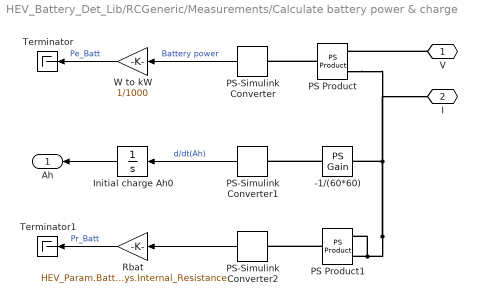
== system HEV_Battery_Det_Lib/RCGeneric/Measurements/Calculate battery power & charge ==
  -1/(60*60) : fl_lib/Physical Signals/Functions/PS Gain  gain=-1/(60*60)
  Initial charge Ah0 : Integrator  InitialCondition=HEV_Param.Battery_Sys.Maximum_Capacity
  PS Product : fl_lib/Physical Signals/Functions/PS Product
      settings: SourceProductName=Simscape
  PS Product1 : fl_lib/Physical Signals/Functions/PS Product
      settings: SourceProductName=Simscape
  PS-Simulink Converter : nesl_utility/PS-Simulink Converter  PhysicalDomain=network_engine_domain  SubClassName=ps_output  LeftPortType=input  RightPortType=output  PseudoPeriodic=off  Frequencies=[]  Unit=W  AffineConversion=off
  PS-Simulink Converter1 : nesl_utility/PS-Simulink Converter  PhysicalDomain=network_engine_domain  SubClassName=ps_output  LeftPortType=input  RightPortType=output  PseudoPeriodic=off  Frequencies=[]  Unit=1  AffineConversion=off
  PS-Simulink Converter2 : nesl_utility/PS-Simulink Converter  PhysicalDomain=network_engine_domain  SubClassName=ps_output  LeftPortType=input  RightPortType=output  PseudoPeriodic=off  Frequencies=[]  Unit=1  AffineConversion=off
  Rbat : Gain  Gain=HEV_Param.Battery_Sys.Internal_Resistance
  Terminator : Terminator
  Terminator1 : Terminator
  W to kW : Gain  Gain=1/1000
  V : PMIOPort  Port=1  Side=Left
  I : PMIOPort  Port=2  Side=Left
  Ah : Outport
  wires:
  Rbat/1 -> Terminator1/1  "Pr_Batt"
  PS-Simulink Converter2/1 -> Rbat/1
  Initial charge Ah0/1 -> Ah/1
  PS-Simulink Converter1/1 -> Initial charge Ah0/1  "d/dt(Ah)"
  W to kW/1 -> Terminator/1  "Pe_Batt"
  PS-Simulink Converter/1 -> W to kW/1  "Battery power"
  connections:
  PS Product1/RConn1 -- PS-Simulink Converter2/LConn1
  -1/(60*60)/RConn1 -- PS-Simulink Converter1/LConn1
  PS Product1/LConn2 -- PS Product1/LConn1 -- -1/(60*60)/LConn1 -- I/RConn1 -- PS Product/LConn2
  V/RConn1 -- PS Product/LConn1
  PS Product/RConn1 -- PS-Simulink Converter/LConn1
